simulink model "controlador_proyecto_simu"  (R2020b)
settings: Solver=VariableStepAuto  StartTime=0.0  StopTime=5  RelTol=1e-3
values from neighbouring files (symbols this model uses):
  p01 = xn(6)    [Algebraico_proyecto.m]
  p11 = xn(5)    [Algebraico_proyecto.m]
  p21 = xn(4)    [Algebraico_proyecto.m]
  q01 = xn(3)    [Algebraico_proyecto.m]
  q11 = xn(2)    [Algebraico_proyecto.m]
  q21 = xn(1)    [Algebraico_proyecto.m]
  Tmd = 0.0746/10    (= 0.00746)    [Algebraico_proyecto.m]    (also in PID_proyecto.m = 0.0047)
settings Model: Creator=KAROL GUACAS  LastModifiedBy=KAROL GUACAS

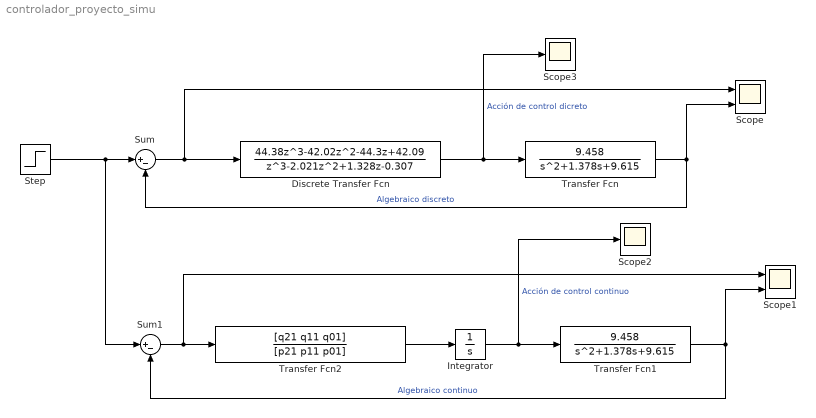
== system controlador_proyecto_simu ==
  Discrete Transfer Fcn : DiscreteTransferFcn  Numerator=[44.38 -42.02 -44.3 42.09]  Denominator=[1 -2.021 1.328 -0.307]  SampleTime=Tmd
  Integrator : Integrator
  Scope : Scope  NumInputPorts=2
  Scope1 : Scope  NumInputPorts=2
  Scope2 : Scope
  Scope3 : Scope
  Step : Step  Time=0  SampleTime=0
  Sum : Sum  Inputs=|+-
  Sum1 : Sum  Inputs=|+-
  Transfer Fcn : TransferFcn  Numerator=[9.458]  Denominator=[1 1.378 9.615]
  Transfer Fcn1 : TransferFcn  Numerator=[9.458]  Denominator=[1 1.378 9.615]
  Transfer Fcn2 : TransferFcn  Numerator=[q21 q11 q01]  Denominator=[p21 p11 p01]
  wires:
  Step/1 -> Sum1/1, Sum/1
  Sum/1 -> Discrete Transfer Fcn/1, Scope/1
  Discrete Transfer Fcn/1 -> Scope3/1, Transfer Fcn/1  "Acción de control dicreto"
  Transfer Fcn/1 -> Scope/2, Sum/2  "Algebraico discreto"
  Transfer Fcn2/1 -> Integrator/1
  Sum1/1 -> Transfer Fcn2/1, Scope1/1
  Transfer Fcn1/1 -> Scope1/2, Sum1/2  "Algebraico continuo"
  Integrator/1 -> Transfer Fcn1/1, Scope2/1  "Acción de control continuo"
